simulink model "sim13b"  (R2015a)
settings: Solver=ode45  StartTime=0.0  StopTime=10.0  RelTol=1e-3
values from neighbouring files (symbols this model uses):
  k1 = 1/yl    (= 20)    [lab2.m]
  k2 = sqrt(2*k1)    [lab2.m]
  yl = 0.05    [lab2.m]
undefined symbols (not defined in the file or in its folder): sgn
libraries: simulink x2
settings Model: Creator=abran  LastModifiedBy=abran

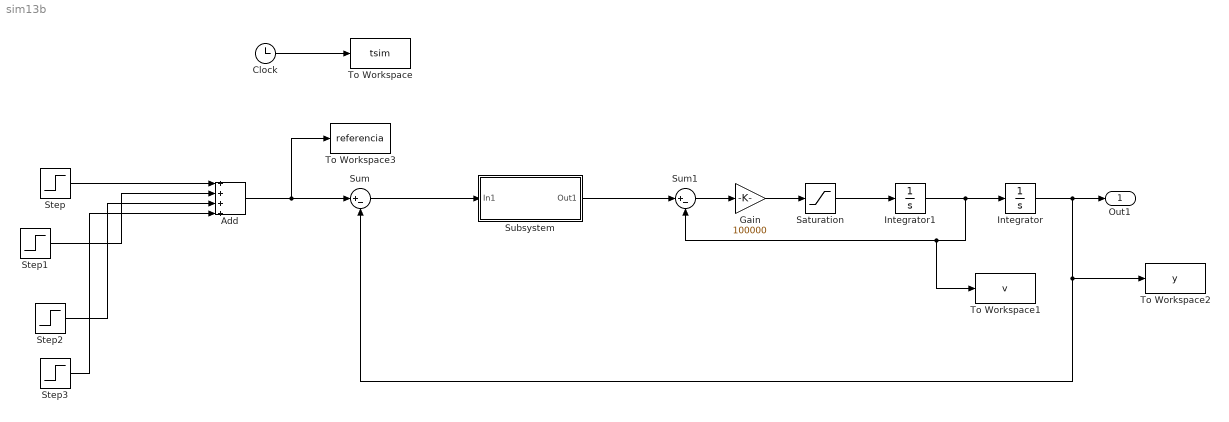
== system sim13b ==
  Add : Sum  Inputs=++++
  Clock : Clock
  Gain : Gain  Gain=100000
  Integrator : Integrator  InitialCondition=1
  Integrator1 : Integrator
  Saturation : Saturate  UpperLimit=1  LowerLimit=-1
  Step : Step  SampleTime=0
  Step1 : Step  Time=5  After=3  SampleTime=0
  Step2 : Step  Time=10  After=-10  SampleTime=0
  Step3 : Step  Time=15  After=10  SampleTime=0
  Subsystem : Subsystem
  Sum : Sum  Inputs=|+-
  Sum1 : Sum  Inputs=|+-
  To Workspace : ToWorkspace  VariableName=tsim  SampleTime=-1
  To Workspace1 : ToWorkspace  VariableName=v  SampleTime=-1
  To Workspace2 : ToWorkspace  VariableName=y  SampleTime=-1
  To Workspace3 : ToWorkspace  VariableName=referencia  SampleTime=-1
  Out1 : Outport
  wires:
  Sum1/1 -> Gain/1
  Gain/1 -> Saturation/1
  Saturation/1 -> Integrator1/1
  Integrator1/1 -> To Workspace1/1, Sum1/2, Integrator/1
  Integrator/1 -> To Workspace2/1, Sum/2, Out1/1
  Clock/1 -> To Workspace/1
  Subsystem/1(Out1) -> Sum1/1
  Sum/1 -> Subsystem/1(In1)
  Add/1 -> To Workspace3/1, Sum/1
  Step/1 -> Add/1
  Step1/1 -> Add/2
  Step2/1 -> Add/3
  Step3/1 -> Add/4

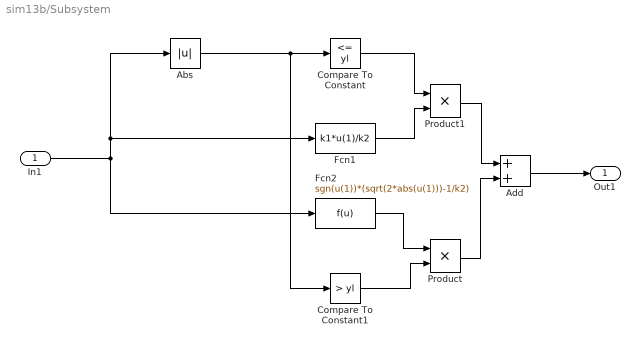
== system sim13b/Subsystem ==
  In1 : Inport
  Abs : Abs
  Add : Sum
  Compare To Constant : simulink/Logic and Bit Operations/Compare To Constant  relop=<=  const=yl  OutDataTypeStr=boolean
  Compare To Constant1 : simulink/Logic and Bit Operations/Compare To Constant  relop=>  const=yl  OutDataTypeStr=boolean
  Fcn1 : Fcn  Expr=k1*u(1)/k2
  Fcn2 : Fcn  Expr=sgn(u(1))*(sqrt(2*abs(u(1)))-1/k2)
  Product : Product
  Product1 : Product
  Out1 : Outport
  wires:
  Product/1 -> Add/2
  Product1/1 -> Add/1
  Compare To Constant/1 -> Product1/1
  Abs/1 -> Compare To Constant1/1, Compare To Constant/1
  Fcn1/1 -> Product1/2
  Fcn2/1 -> Product/1
  Compare To Constant1/1 -> Product/2
  Add/1 -> Out1/1
  In1/1 -> Fcn2/1, Fcn1/1, Abs/1
